simulink model "Automatic_Trans_Controller"  (R2020a)
settings: Solver=VariableStepAuto  StartTime=0.0  StopTime=10.0  RelTol=1e-3
values from neighbouring files (symbols this model uses):
  EMAP = -40.0 215.0 245.0 264.0 264.0 267.0 267.0 267.0 267.0 267.0 -44.0 117.0 208.0 260.0 279.0 290.0 297.0 301.0 301.0 301.0 -49.0 85.0 178.0 241.0 282.0 293.0 305.0 308.0 312.0 312.0 -53.0 66.0 148.0 219.0 275.0 297.0 305.0 312.0 319.0 319.0 -57.0 44.0 122.0 193.0 260.0 290.0 305.0 319.0 327.0 327.0 -61.0 29.0 104.0 167.0 238.0 275.0 301.0 323.0 327.0 334.0 -65.0 10.0 85.0 152.0 223.0 260.0 293.0 319.    [Data_Dictionary.sldd]
  Iei = 0.021991488283555904    [Data_Dictionary.sldd]
  NE_VEC = 799.99999999999989 1200.0 1599.9999999999998 1999.9999999999998 2400.0 2800.0000000000005 3199.9999999999995 3599.9999999999995 3999.9999999999995 4400.0 4800.0    [Data_Dictionary.sldd]
  TH_VEC = 0.0 20.0 30.0 40.0 50.0 60.0 70.0 80.0 90.0 100.0    [Data_Dictionary.sldd]
settings Model: DataDictionary=Data_Dictionary.sldd  OrderedModelArguments=off  Creator=Shivam  LastModifiedBy=Shivam

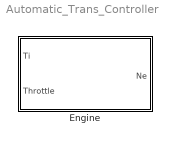
== system Automatic_Trans_Controller ==
  Engine : Subsystem

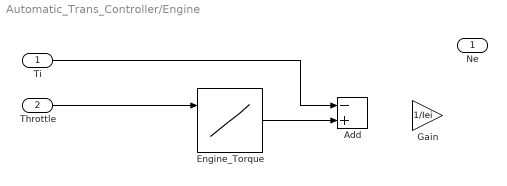
== system Automatic_Trans_Controller/Engine ==
  Ti : Inport
  Throttle : Inport  Port=2
  Add : Sum  Inputs=-+
  Engine_Torque : Lookup_n-D  BreakpointsForDimension1=TH_VEC  BreakpointsForDimension2=NE_VEC  Table=EMAP  InternalRulePriority=Speed  RndMeth=Simplest  InputSameDT=on
  Gain : Gain  Gain=1/Iei
  Ne : Outport
  wires:
  Ti/1 -> Add/1
  Engine_Torque/1 -> Add/2
  Throttle/1 -> Engine_Torque/1
